simulink model "ca_interp"  (R2023b)
settings: Solver=VariableStepDiscrete  StartTime=0.0  StopTime=DUC_LINEUP_param.endTime  RelTol=1e-3  EnableMultiTasking=on
PreLoadFcn:
  | % Run the setup script when the model is opened
  | setup_ca_interp;
InitFcn:
  | % Run the setup script again just before the
  | % model is run, so that any updates made
  | % after opening are applied.
  | 
  | setup_ca_interp;
StopFcn:
  | ca_interp_output_analysis;
values from neighbouring files (symbols this model uses):
  DUC_SUMMER_multiplication_factor = 1    [setup_ca_interp.m]
  DUC_SUMMER_Number_of_bits_to_shift_left = 0    [setup_ca_interp.m]
undefined symbols (not defined in the file or in its folder): AdvDSPBChannelOutDisplay, AdvDSPBDMemDisplay, dpoly, dspba_ChannelInVis, dspba_ChannelOutVis, dspba_internal_get_channel_ports, DUC_LINEUP_param, evalAionMaskParam, latency, primtype, UseDontCare, value
libraries: DSPBAPrim x53, simulink x18, DSPBAModelBus x14, DSPBABase x12, DSPBAFilters x2
(part 1 of 2)
Description:
  | DSP Builder Advanced Template for Template Design implementing ModelIP designs
settings Model: Creator=mjervis  LastModifiedBy=5g
settings SolverCC: AlgebraicLoopSolver=TrustRegion
settings DataIOCC: LimitDataPoints=on  SaveFormat=Array  SignalLoggingSaveFormat=ModelDataLogs  ReturnWorkspaceOutputs=off
settings OptimizationCC: ExpressionDepthLimit=2147483647  LifeSpan=inf
settings DebuggingCC: UnderspecifiedInitializationDetection=Classic  MergeDetectMultiDrivingBlocksExec=none  SolverPrmCheckMsg=warning  InheritedTsInSrcMsg=none  IntegerOverflowMsg=none  FcnCallInpInsideContextMsg=warning  UnconnectedInputMsg=warning  UnconnectedOutputMsg=warning  UnconnectedLineMsg=warning  StateNameClashWarn=warning  SFUnexpectedBacktrackingDiag=warning  SFNoUnconditionalDefaultTransitionDiag=warning  SFExecutionAtInitializationDiag=none  IntegerSaturationMsg=none  ArithmeticOperatorsInVariantConditions=warning
settings HardwareCC: ProdBitPerPointer=32  ProdBitPerSizeT=32  ProdBitPerPtrDiffT=32  ProdLargestAtomicFloat=None  ProdIntDivRoundTo=Undefined  ProdEndianess=Unspecified  ProdWordSize=32  ProdHWDeviceType=32-bit Generic
settings ModelReferenceCC: EnableRefExpFcnMdlSchedulingChecks=on  PropagateSignalLabelsOutOfModel=off
settings SFSimCC: SimUseLocalCustomCode=off  CustomCodeUndefinedFunction=UseInterfaceOnly
settings RTWCC: RTWUseLocalCustomCode=off  DLArmComputeVersion=19.05
settings CodeAppCC: StateflowObjectComments=on
settings GRTTargetCC: TargetLangStandard=C89/C90 (ANSI)  CombineOutputUpdateFcns=off  GRTInterface=on
settings ConfigComp: CovMetricSettings=dw  CovSaveCumulativeToWorkspaceVar=on  CovSaveSingleToWorkspaceVar=on  CovExternalEMLEnable=off

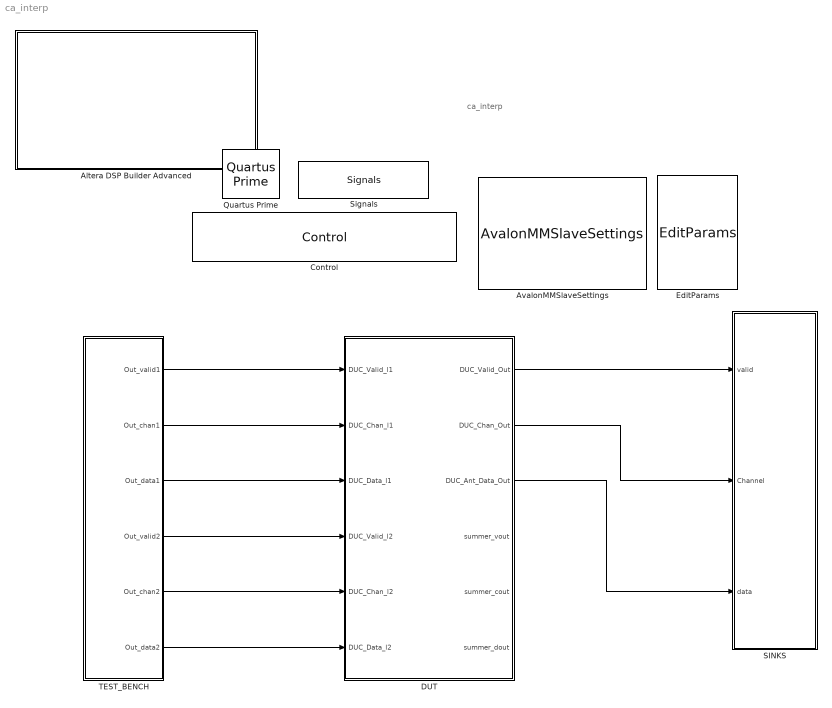
== system ca_interp ==
  note: ca_interp
  Altera DSP Builder Advanced : Subsystem  mask(DSP Builder Advanced Blockset Ignored Block){}
      settings: OpenFcn=web('http://www.altera.com', '-new');
      mask Display: image(imread('intellogo.tif'));
  AvalonMMSlaveSettings : DSPBABase/AvalonMMSlaveSettings
  Control : DSPBABase/Control  generate=on  language=VHDL  destination=./rtl  destination_gui=./rtl  make_full_path=off  path_is_relative=on  autotestbench=on  signaldepth=2  coveragetestbench=off  logs=off  spacewidth=2  spacenum=1  addrwidth=10  datawidth=16  dataendian=Big Endian  hierarchicalnames=off  ramThresholdBits=-1  distRamThresholdBits=-1  mlabThresholdBits=-1  hardMultiplierThresholdLuts=-1  version=20150801  errorOnChanMismatch=1  errorOnGPIOMismatch=0  importModelsimResults=0  cycleAccurate=off  reinterpretCastMult=off  paramFile=ca_interp_params.xml
  DUT : Subsystem
  EditParams : DSPBABase/EditParams  version=20090407
  Quartus Prime : DSPBABase/Quartus Prime  version=20090407
  SINKS : Subsystem
  Signals : DSPBABase/Signals  clk=clk  freq=240  margin=0  rst=areset  rstactive=High  bus=bus  enbusclock=off  busfreq=491.52  bussync=off  version=20090407
  TEST_BENCH : Subsystem
  wires:
  DUT/1(DUC_Valid_Out) -> SINKS/1(valid)
  DUT/3(DUC_Ant_Data_Out) -> SINKS/3(data)
  DUT/2(DUC_Chan_Out) -> SINKS/2(Channel)
  TEST_BENCH/1(Out_valid1) -> DUT/1(DUC_Valid_l1)
  TEST_BENCH/2(Out_chan1) -> DUT/2(DUC_Chan_l1)
  TEST_BENCH/3(Out_data1) -> DUT/3(DUC_Data_l1)
  TEST_BENCH/4(Out_valid2) -> DUT/4(DUC_Valid_l2)
  TEST_BENCH/5(Out_chan2) -> DUT/5(DUC_Chan_l2)
  TEST_BENCH/6(Out_data2) -> DUT/6(DUC_Data_l2)

== system ca_interp/Altera DSP Builder Advanced ==

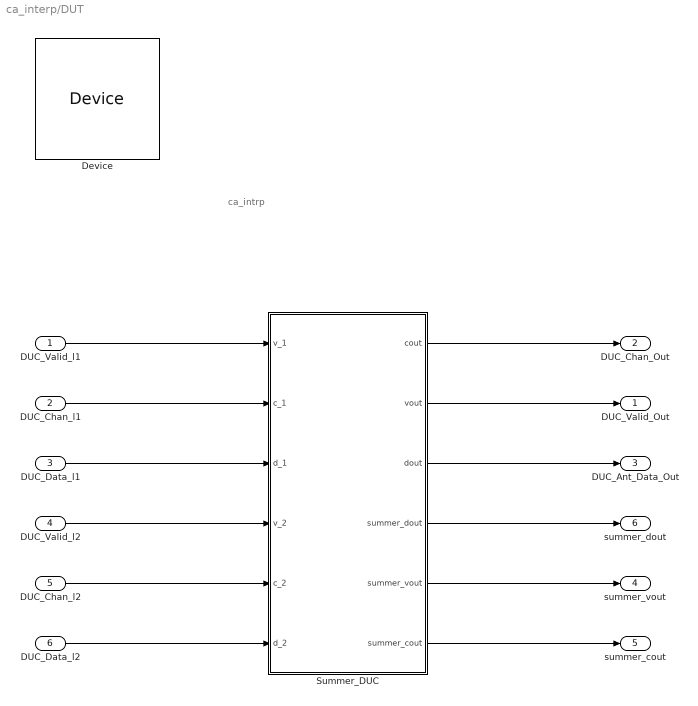
== system ca_interp/DUT ==
  note: ca_intrp
  DUC_Valid_l1 : Inport
  DUC_Chan_l1 : Inport  Port=2
  DUC_Data_l1 : Inport  Port=3
  DUC_Valid_l2 : Inport  Port=4
  DUC_Chan_l2 : Inport  Port=5
  DUC_Data_l2 : Inport  Port=6
  Device : DSPBABase/Device  family=Arria 10  deviceMember=Stratix V GX  stratix4device=Stratix IV GX  hardcopy4device=HardCopy IV E  stratix5device=Stratix V GX  device=10AS066N2F40I1SGES  speed=1  stratixSpeed=-5  stratix2Speed=-3  stratix3Speed=-3  stratix4gxSpeed=-2  stratix4gtSpeed=-1  cyclone2Speed=-6  cyclone3Speed=-7  arria2Speed=-4  cyclone4eSpeed=-8  stratix5Speed=-3  arria5Speed=-4  arriaSpeed=-6  cyclone3lsSpeed=-7  cyclone5Speed=-6  arria2gzSpeed=-3  nightFurySpeed=-2  ecp2Speed=-7  hardcopycompat=off  version=20140217  max10flashmode=off  max10nomeminit=off
  Summer_DUC : Subsystem
  DUC_Valid_Out : Outport
  DUC_Chan_Out : Outport  Port=2
  DUC_Ant_Data_Out : Outport  Port=3
  summer_vout : Outport  Port=4
  summer_cout : Outport  Port=5
  summer_dout : Outport  Port=6
  wires:
  DUC_Valid_l2/1 -> Summer_DUC/4(v_2)
  DUC_Chan_l2/1 -> Summer_DUC/5(c_2)
  DUC_Data_l2/1 -> Summer_DUC/6(d_2)
  DUC_Valid_l1/1 -> Summer_DUC/1(v_1)
  DUC_Chan_l1/1 -> Summer_DUC/2(c_1)
  DUC_Data_l1/1 -> Summer_DUC/3(d_1)
  Summer_DUC/3(dout) -> DUC_Ant_Data_Out/1
  Summer_DUC/2(vout) -> DUC_Valid_Out/1
  Summer_DUC/1(cout) -> DUC_Chan_Out/1
  Summer_DUC/4(summer_dout) -> summer_dout/1
  Summer_DUC/5(summer_vout) -> summer_vout/1
  Summer_DUC/6(summer_cout) -> summer_cout/1

== system ca_interp/SINKS ==
  valid : Inport
  Channel : Inport  Port=2
  data : Inport  Port=3
  ChanView : DSPBABase/ChanView  nchans=8  chan_vector=[0:7]  outsvalid=off  latency=1  version=20090407
  ChanView1 : DSPBABase/ChanView  nchans=8  chan_vector=[0:7]  outsvalid=off  latency=1  version=20090407
  Complex to Real-Imag2 : ComplexToRealImag
  ImagScope : Scope  NumInputPorts=8
  RealScope : Scope  NumInputPorts=8
  Scope : Scope  NumInputPorts=3
  To Workspace : ToWorkspace  Commented=on  VariableName=DUC_Ant_Data_out  SaveFormat=Timeseries  SampleTime=-1
  To Workspace1 : ToWorkspace  Commented=on  VariableName=DUC_Ant_Data_vout  SaveFormat=Timeseries  SampleTime=-1
  TraceAntennaData : Subsystem  Commented=on  TreatAsAtomicUnit=on
  TraceAntennaData1 : Subsystem  TreatAsAtomicUnit=on
  dataScope : Scope  NumInputPorts=2
  wires:
  Complex to Real-Imag2/1 -> dataScope/1, ChanView/1
  Channel/1 -> TraceAntennaData1/2(ChIn), Scope/2, ChanView1/3, ChanView/3
  Complex to Real-Imag2/2 -> dataScope/2, ChanView1/1
  ChanView1/2 -> ImagScope/2
  ChanView1/3 -> ImagScope/3
  ChanView1/4 -> ImagScope/4
  ChanView1/1 -> ImagScope/1
  ChanView/3 -> RealScope/3
  ChanView/1 -> RealScope/1
  ChanView/4 -> RealScope/4
  ChanView/2 -> RealScope/2
  ChanView/5 -> RealScope/5
  ChanView/6 -> RealScope/6
  ChanView/7 -> RealScope/7
  ChanView/8 -> RealScope/8
  ChanView1/5 -> ImagScope/5
  ChanView1/6 -> ImagScope/6
  ChanView1/7 -> ImagScope/7
  ChanView1/8 -> ImagScope/8
  valid/1 -> TraceAntennaData1/Enable, To Workspace1/1, Scope/1, TraceAntennaData/Enable, ChanView1/2, ChanView/2
  data/1 -> TraceAntennaData1/1(DataIn), To Workspace/1, Scope/3, TraceAntennaData/1(DataIn), Complex to Real-Imag2/1

== system ca_interp/TEST_BENCH ==
  Data Type Conversion : DataTypeConversion  OutDataTypeStr=uint8  SaturateOnIntegerOverflow=off  RndMeth=Floor
  Repeating Sequence channel : simulink/Sources/Repeating Sequence Stair  OutValues=DUC_LINEUP_param.duc_channel  tsamp=1  OutMin=[]  OutMax=[]  OutDataTypeStr=uint8  OutputDataTypeScalingMode=uint8  OutDataType=fixdt(1,16)  ConRadixGroup=Best Precision: Vector-wise  OutScaling=[]
  Repeating Sequence valid : simulink/Sources/Repeating Sequence Stair  OutValues=DUC_LINEUP_param.duc_valid  tsamp=1  OutMin=[]  OutMax=[]  OutDataTypeStr=fixdt('boolean')  OutputDataTypeScalingMode=Specify via dialog  OutDataType=fixdt('boolean')  ConRadixGroup=Best Precision: Vector-wise  OutScaling=[]
  Subsystem1 : Subsystem
  Subsystem2 : Subsystem
  Out_valid1 : Outport
  Out_chan1 : Outport  Port=2
  Out_data1 : Outport  Port=3
  Out_valid2 : Outport  Port=4
  Out_chan2 : Outport  Port=5
  Out_data2 : Outport  Port=6
  wires:
  Repeating Sequence valid/1 -> Out_valid2/1, Out_valid1/1  "valid signal"
  Repeating Sequence channel/1 -> Data Type Conversion/1  "channel count signal"
  Data Type Conversion/1 -> Out_chan2/1, Out_chan1/1
  Subsystem1/1(Out_data1) -> Out_data1/1
  Subsystem2/1(Out_data2) -> Out_data2/1

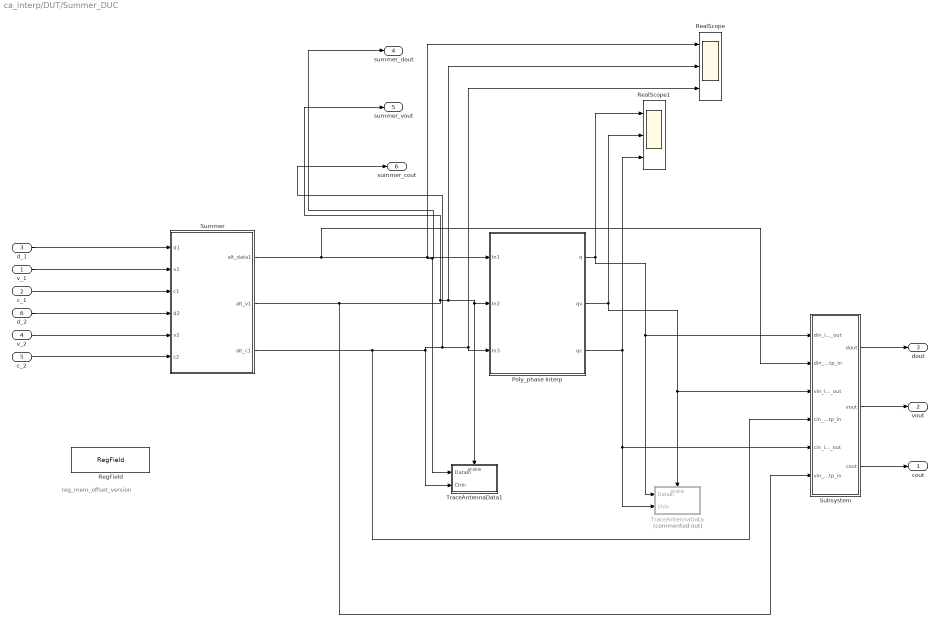
== system ca_interp/DUT/Summer_DUC ==
  note: reg_mem_offset_version
  v_1 : Inport
  c_1 : Inport  Port=2
  d_1 : Inport  Port=3
  v_2 : Inport  Port=4
  c_2 : Inport  Port=5
  d_2 : Inport  Port=6
  Poly_phase Interp : Subsystem
  RealScope : Scope  NumInputPorts=3
  RealScope1 : Scope  NumInputPorts=3
  RegField : DSPBAModelBus/RegField  reg_name=DUC_LINEUP_param.reg_version.mem_offset  reg_rwmode=Read/Write  reg_msb=31  reg_lsb=0  reg_mode=Specify via dialog  reg_type=ufix(32)  reg_scale=2^0  reg_init=DUC_LINEUP_param.reg_version.Version_reg_val  reg_desc=Version_Output  reg_modal=off  reg_desc0=0  reg_desc1=0  reg_desc2=0  reg_desc3=0  reg_desc4=0  reg_desc5=0  reg_desc6=0  reg_desc7=0  reg_addr=13  SampleTime=-1  version=20090407
  Subsystem : Subsystem
  Summer : Subsystem  mask{ClockMargin=DUC_LINEUP_param.ClockMargin, output_word_length=DUC_LINEUP_param.output_word_length, output_fraction_length=DUC_LINEUP_param.output_fraction_length, Summer_Multiplication_fact=DUC_SUMMER_multiplication_factor, Summer_left_shift_fact=DUC_SUMMER_Number_of_bits_to_shift_left, Pipeline_stages=2}
      mask Display:
      | disp('SUMMER');
      | port_label('input',1,'d0');
      | port_label('input',2,'v0');
      | port_label('input',3,'c0');
      | 
      | port_label('input',4,'d1');
      | port_label('input',5,'v1');
      | port_label('input',6,'c1');
      | 
      | 
      | port_label('output',1,'q');
      | port_label('output',2,'q_v');
      | port_label('output',3,'q_c');
  TraceAntennaData : Subsystem  Commented=on  TreatAsAtomicUnit=on
  TraceAntennaData1 : Subsystem  TreatAsAtomicUnit=on
  cout : Outport
  vout : Outport  Port=2
  dout : Outport  Port=3
  summer_dout : Outport  Port=4
  summer_vout : Outport  Port=5
  summer_cout : Outport  Port=6
  wires:
  c_1/1 -> Summer/3(c1)
  d_2/1 -> Summer/4(d2)
  v_2/1 -> Summer/5(v2)
  c_2/1 -> Summer/6(c2)
  v_1/1 -> Summer/2(v1)
  d_1/1 -> Summer/1(d1)
  Summer/2(alt_v1) -> Subsystem/6(vin_intp_in), summer_vout/1, TraceAntennaData1/Enable, Poly_phase Interp/2(In2), RealScope/2
  Summer/3(alt_c1) -> Subsystem/4(cin_intp_in), summer_cout/1, RealScope/3, Poly_phase Interp/3(In3), TraceAntennaData1/2(ChIn)
  Poly_phase Interp/1(q) -> RealScope1/1, TraceAntennaData/1(DataIn), Subsystem/1(din_intp_out)
  Poly_phase Interp/2(qv) -> RealScope1/2, Subsystem/3(vin_intp_out), TraceAntennaData/Enable
  Poly_phase Interp/3(qc) -> RealScope1/3, TraceAntennaData/2(ChIn), Subsystem/5(cin_intp_out)
  Summer/1(alt_data1) -> RealScope/1, Poly_phase Interp/1(In1), summer_dout/1, TraceAntennaData1/1(DataIn), Subsystem/2(din_intp_in)
  Subsystem/1(dout) -> dout/1
  Subsystem/2(vout) -> vout/1
  Subsystem/3(cout) -> cout/1

== system ca_interp/SINKS/TraceAntennaData ==
  DataIn : Inport
  Enable : EnablePort
  DucAntDataOut : ToWorkspace  VariableName=DUC_Ant_Data_Out  SaveFormat=Timeseries  SampleTime=-1
  wires:
  DataIn/1 -> DucAntDataOut/1

== system ca_interp/SINKS/TraceAntennaData1 ==
  DataIn : Inport
  ChIn : Inport  Port=2
  Enable : EnablePort
  DucAntDataOut : ToWorkspace  VariableName=PolyPhase0_dOut  SampleTime=-1
  DucAntDataOut1 : ToWorkspace  VariableName=PolyPhase0_cOut  SampleTime=-1
  wires:
  DataIn/1 -> DucAntDataOut/1
  ChIn/1 -> DucAntDataOut1/1

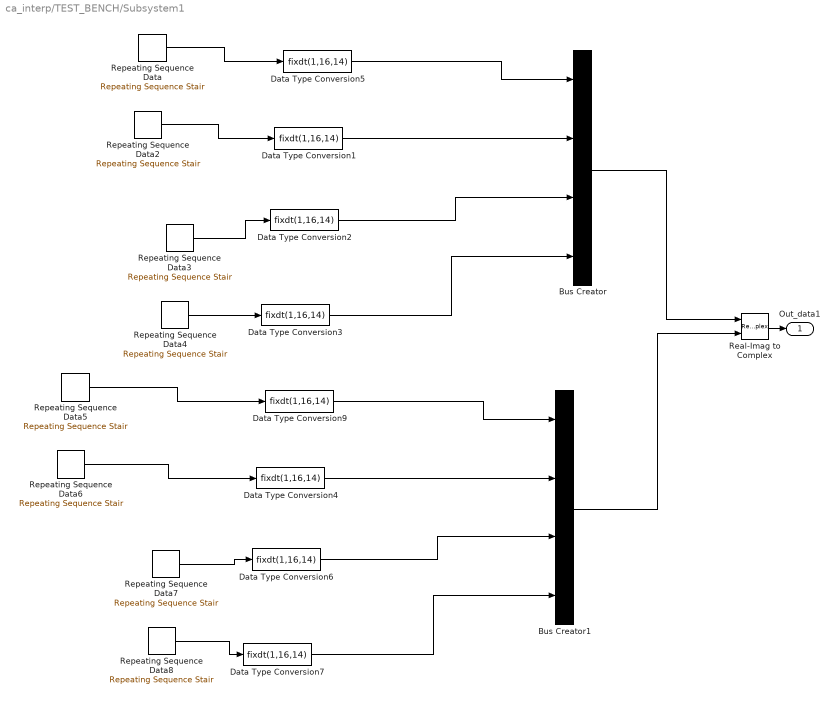
== system ca_interp/TEST_BENCH/Subsystem1 ==
  Bus Creator : BusCreator  Inputs=4
  Bus Creator1 : BusCreator  Inputs=4
  Data Type Conversion{1..7,9} (8 alike) : DataTypeConversion  OutDataTypeStr=fixdt(1,16,14)  SaturateOnIntegerOverflow=off  RndMeth=Floor
  Real-Imag to Complex : RealImagToComplex
  Repeating Sequence Data : simulink/Sources/Repeating Sequence Stair  OutValues=real(DUC_LINEUP_param.inputdata_l1(:,1))  tsamp=1  OutMin=[]  OutMax=[]  OutDataTypeStr=fixdt(1,16)  OutputDataTypeScalingMode=Specify via dialog  OutDataType=fixdt(1,16)  ConRadixGroup=Best Precision: Vector-wise  OutScaling=[]
  Repeating Sequence Data2 : simulink/Sources/Repeating Sequence Stair  OutValues=real(DUC_LINEUP_param.inputdata_l1(:,2))  tsamp=1  OutMin=[]  OutMax=[]  OutDataTypeStr=fixdt(1,16)  OutputDataTypeScalingMode=Specify via dialog  OutDataType=fixdt(1,16)  ConRadixGroup=Best Precision: Vector-wise  OutScaling=[]
  Repeating Sequence Data3 : simulink/Sources/Repeating Sequence Stair  OutValues=real(DUC_LINEUP_param.inputdata_l1(:,3))  tsamp=1  OutMin=[]  OutMax=[]  OutDataTypeStr=fixdt(1,16)  OutputDataTypeScalingMode=Specify via dialog  OutDataType=fixdt(1,16)  ConRadixGroup=Best Precision: Vector-wise  OutScaling=[]
  Repeating Sequence Data4 : simulink/Sources/Repeating Sequence Stair  OutValues=real(DUC_LINEUP_param.inputdata_l1(:,4))  tsamp=1  OutMin=[]  OutMax=[]  OutDataTypeStr=fixdt(1,16)  OutputDataTypeScalingMode=Specify via dialog  OutDataType=fixdt(1,16)  ConRadixGroup=Best Precision: Vector-wise  OutScaling=[]
  Repeating Sequence Data5 : simulink/Sources/Repeating Sequence Stair  OutValues=imag(DUC_LINEUP_param.inputdata_l1(:,1))  tsamp=1  OutMin=[]  OutMax=[]  OutDataTypeStr=fixdt(1,16)  OutputDataTypeScalingMode=Specify via dialog  OutDataType=fixdt(1,16)  ConRadixGroup=Best Precision: Vector-wise  OutScaling=[]
  Repeating Sequence Data6 : simulink/Sources/Repeating Sequence Stair  OutValues=imag(DUC_LINEUP_param.inputdata_l1(:,2))  tsamp=1  OutMin=[]  OutMax=[]  OutDataTypeStr=fixdt(1,16)  OutputDataTypeScalingMode=Specify via dialog  OutDataType=fixdt(1,16)  ConRadixGroup=Best Precision: Vector-wise  OutScaling=[]
  Repeating Sequence Data7 : simulink/Sources/Repeating Sequence Stair  OutValues=imag(DUC_LINEUP_param.inputdata_l1(:,3))  tsamp=1  OutMin=[]  OutMax=[]  OutDataTypeStr=fixdt(1,16)  OutputDataTypeScalingMode=Specify via dialog  OutDataType=fixdt(1,16)  ConRadixGroup=Best Precision: Vector-wise  OutScaling=[]
  Repeating Sequence Data8 : simulink/Sources/Repeating Sequence Stair  OutValues=imag(DUC_LINEUP_param.inputdata_l1(:,4))  tsamp=1  OutMin=[]  OutMax=[]  OutDataTypeStr=fixdt(1,16)  OutputDataTypeScalingMode=Specify via dialog  OutDataType=fixdt(1,16)  ConRadixGroup=Best Precision: Vector-wise  OutScaling=[]
  Out_data1 : Outport
  wires:
  Data Type Conversion6/1 -> Bus Creator1/3
  Bus Creator1/1 -> Real-Imag to Complex/2
  Repeating Sequence Data/1 -> Data Type Conversion5/1
  Data Type Conversion3/1 -> Bus Creator/4
  Repeating Sequence Data8/1 -> Data Type Conversion7/1
  Data Type Conversion5/1 -> Bus Creator/1
  Real-Imag to Complex/1 -> Out_data1/1
  Repeating Sequence Data2/1 -> Data Type Conversion1/1
  Bus Creator/1 -> Real-Imag to Complex/1
  Data Type Conversion9/1 -> Bus Creator1/1
  Data Type Conversion1/1 -> Bus Creator/2
  Repeating Sequence Data3/1 -> Data Type Conversion2/1
  Repeating Sequence Data7/1 -> Data Type Conversion6/1
  Repeating Sequence Data4/1 -> Data Type Conversion3/1
  Repeating Sequence Data6/1 -> Data Type Conversion4/1
  Data Type Conversion2/1 -> Bus Creator/3
  Repeating Sequence Data5/1 -> Data Type Conversion9/1
  Data Type Conversion7/1 -> Bus Creator1/4
  Data Type Conversion4/1 -> Bus Creator1/2

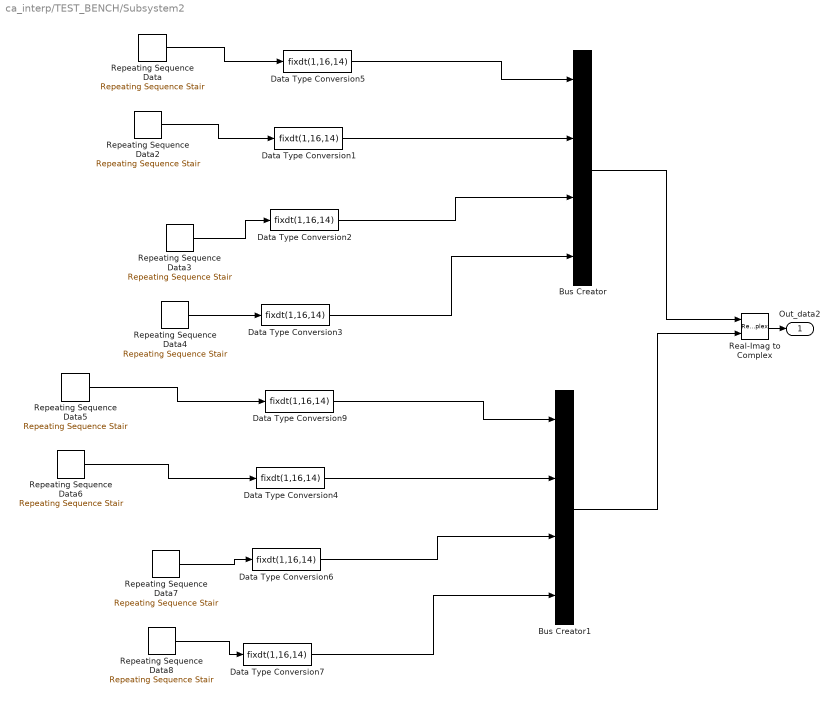
== system ca_interp/TEST_BENCH/Subsystem2 ==
  Bus Creator : BusCreator  Inputs=4
  Bus Creator1 : BusCreator  Inputs=4
  Data Type Conversion{1..7,9} (8 alike) : DataTypeConversion  OutDataTypeStr=fixdt(1,16,14)  SaturateOnIntegerOverflow=off  RndMeth=Floor
  Real-Imag to Complex : RealImagToComplex
  Repeating Sequence Data : simulink/Sources/Repeating Sequence Stair  OutValues=real(DUC_LINEUP_param.inputdata_l2(:,1))  tsamp=1  OutMin=[]  OutMax=[]  OutDataTypeStr=fixdt(1,16)  OutputDataTypeScalingMode=Specify via dialog  OutDataType=fixdt(1,16)  ConRadixGroup=Best Precision: Vector-wise  OutScaling=[]
  Repeating Sequence Data2 : simulink/Sources/Repeating Sequence Stair  OutValues=real(DUC_LINEUP_param.inputdata_l2(:,2))  tsamp=1  OutMin=[]  OutMax=[]  OutDataTypeStr=fixdt(1,16)  OutputDataTypeScalingMode=Specify via dialog  OutDataType=fixdt(1,16)  ConRadixGroup=Best Precision: Vector-wise  OutScaling=[]
  Repeating Sequence Data3 : simulink/Sources/Repeating Sequence Stair  OutValues=real(DUC_LINEUP_param.inputdata_l2(:,3))  tsamp=1  OutMin=[]  OutMax=[]  OutDataTypeStr=fixdt(1,16)  OutputDataTypeScalingMode=Specify via dialog  OutDataType=fixdt(1,16)  ConRadixGroup=Best Precision: Vector-wise  OutScaling=[]
  Repeating Sequence Data4 : simulink/Sources/Repeating Sequence Stair  OutValues=real(DUC_LINEUP_param.inputdata_l2(:,4))  tsamp=1  OutMin=[]  OutMax=[]  OutDataTypeStr=fixdt(1,16)  OutputDataTypeScalingMode=Specify via dialog  OutDataType=fixdt(1,16)  ConRadixGroup=Best Precision: Vector-wise  OutScaling=[]
  Repeating Sequence Data5 : simulink/Sources/Repeating Sequence Stair  OutValues=imag(DUC_LINEUP_param.inputdata_l2(:,1))  tsamp=1  OutMin=[]  OutMax=[]  OutDataTypeStr=fixdt(1,16)  OutputDataTypeScalingMode=Specify via dialog  OutDataType=fixdt(1,16)  ConRadixGroup=Best Precision: Vector-wise  OutScaling=[]
  Repeating Sequence Data6 : simulink/Sources/Repeating Sequence Stair  OutValues=imag(DUC_LINEUP_param.inputdata_l2(:,2))  tsamp=1  OutMin=[]  OutMax=[]  OutDataTypeStr=fixdt(1,16)  OutputDataTypeScalingMode=Specify via dialog  OutDataType=fixdt(1,16)  ConRadixGroup=Best Precision: Vector-wise  OutScaling=[]
  Repeating Sequence Data7 : simulink/Sources/Repeating Sequence Stair  OutValues=imag(DUC_LINEUP_param.inputdata_l2(:,3))  tsamp=1  OutMin=[]  OutMax=[]  OutDataTypeStr=fixdt(1,16)  OutputDataTypeScalingMode=Specify via dialog  OutDataType=fixdt(1,16)  ConRadixGroup=Best Precision: Vector-wise  OutScaling=[]
  Repeating Sequence Data8 : simulink/Sources/Repeating Sequence Stair  OutValues=imag(DUC_LINEUP_param.inputdata_l2(:,4))  tsamp=1  OutMin=[]  OutMax=[]  OutDataTypeStr=fixdt(1,16)  OutputDataTypeScalingMode=Specify via dialog  OutDataType=fixdt(1,16)  ConRadixGroup=Best Precision: Vector-wise  OutScaling=[]
  Out_data2 : Outport
  wires:
  Data Type Conversion4/1 -> Bus Creator1/2
  Data Type Conversion7/1 -> Bus Creator1/4
  Repeating Sequence Data5/1 -> Data Type Conversion9/1
  Data Type Conversion2/1 -> Bus Creator/3
  Repeating Sequence Data6/1 -> Data Type Conversion4/1
  Repeating Sequence Data4/1 -> Data Type Conversion3/1
  Repeating Sequence Data7/1 -> Data Type Conversion6/1
  Repeating Sequence Data3/1 -> Data Type Conversion2/1
  Data Type Conversion1/1 -> Bus Creator/2
  Data Type Conversion9/1 -> Bus Creator1/1
  Bus Creator/1 -> Real-Imag to Complex/1
  Repeating Sequence Data2/1 -> Data Type Conversion1/1
  Real-Imag to Complex/1 -> Out_data2/1
  Data Type Conversion5/1 -> Bus Creator/1
  Repeating Sequence Data8/1 -> Data Type Conversion7/1
  Data Type Conversion3/1 -> Bus Creator/4
  Repeating Sequence Data/1 -> Data Type Conversion5/1
  Bus Creator1/1 -> Real-Imag to Complex/2
  Data Type Conversion6/1 -> Bus Creator1/3

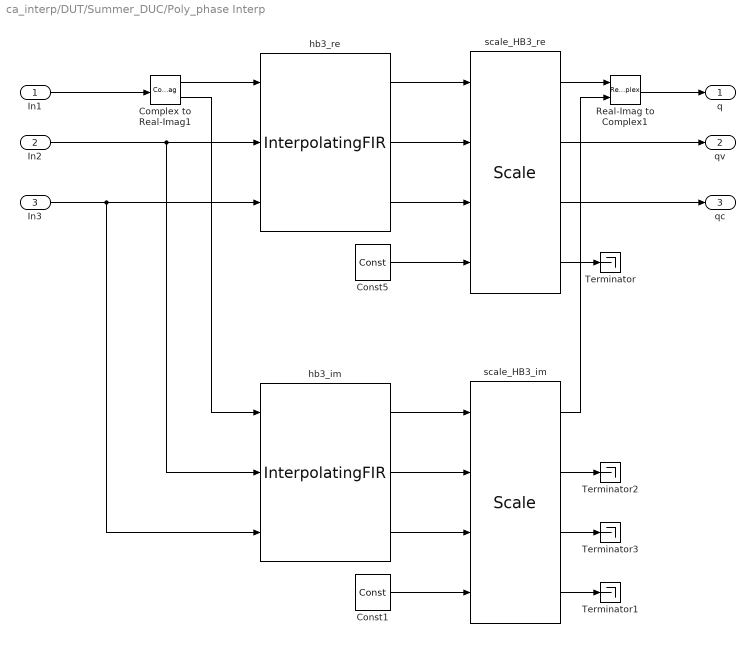
== system ca_interp/DUT/Summer_DUC/Poly_phase Interp ==
  In1 : Inport
  In2 : Inport  Port=2
  In3 : Inport  Port=3
  Complex to Real-Imag1 : ComplexToRealImag
  Const1 : DSPBAPrim/Const  primtype=const  nInputs=0  nOutputs=1  omode=Inherit via internal rule  otype=sfix(16)  scale=2^-15  rndmethod=Unbiased  factor=1  satmethod=Symmetric  shift_vec=[0 1 2 -1]  value=0  inPortNames=['+'; '+';]  outPortNames=[' ']  dspbaimage=dspba_prim.svg  text=fprintf('%s', num2str(value));  style=Optimised  visibilities=8 + 1024  floatPrecision=float32_m23  warnSaturation=on  version=20211007  SampleTime=inf
  Const5 : DSPBAPrim/Const  primtype=const  nInputs=0  nOutputs=1  omode=Inherit via internal rule  otype=sfix(16)  scale=2^-15  rndmethod=Unbiased  factor=1  satmethod=Symmetric  shift_vec=[0 1 2 -1]  value=0  inPortNames=['+'; '+';]  outPortNames=[' ']  dspbaimage=dspba_prim.svg  text=fprintf('%s', num2str(value));  style=Optimised  visibilities=8 + 1024  floatPrecision=float32_m23  warnSaturation=on  version=20211007  SampleTime=inf
  Real-Imag to Complex1 : RealImagToComplex
  Terminator{,1..3} (4 alike) : Terminator
  hb3_im : DSPBAFilters/InterpolatingFIR  nInputRate=491.52  interp=2  nchan=DUC_LINEUP_param.ChanCount  symmetry=Symmetrical  coef=DUC_LINEUP_param.HB_filt3.coeffs  addr=DUC_LINEUP_param.HB_filt6.base_addr_l3  rwmode=Constant  nband=Half Band  exposebus=off  latency=5  version=20090407  recon=off  MM=[0,1,2,3,4,5,6,7,8,9,10,11,12,13,14,15]  resetrezero=off  sharecoef=auto  simulationMode=Standard
  hb3_re : DSPBAFilters/InterpolatingFIR  nInputRate=491.52  interp=2  nchan=DUC_LINEUP_param.ChanCount  symmetry=Symmetrical  coef=DUC_LINEUP_param.HB_filt3.coeffs  addr=DUC_LINEUP_param.HB_filt6.base_addr_l3  rwmode=Constant  nband=Half Band  exposebus=off  latency=5  version=20090407  recon=off  MM=[0,1,2,3,4,5,6,7,8,9,10,11,12,13,14,15]  resetrezero=off  sharecoef=auto  simulationMode=Standard
  scale_HB3_im : DSPBABase/Scale  otype=sfix(DUC_LINEUP_param.output_word_length)  scale=2^-DUC_LINEUP_param.output_fraction_length  rndmethod=Biased  factor=1  satmethod=None  shift_vec=1  latency=2  simulationMode=Use Global Value  version=20090407
  scale_HB3_re : DSPBABase/Scale  otype=sfix(DUC_LINEUP_param.output_word_length)  scale=2^-DUC_LINEUP_param.output_fraction_length  rndmethod=Biased  factor=1  satmethod=None  shift_vec=1  latency=2  simulationMode=Use Global Value  version=20090407
  q : Outport
  qv : Outport  Port=2
  qc : Outport  Port=3
  wires:
  scale_HB3_im/4 -> Terminator1/1
  In3/1 -> hb3_im/3, hb3_re/3
  Complex to Real-Imag1/1 -> hb3_re/1
  hb3_im/1 -> scale_HB3_im/1
  Complex to Real-Imag1/2 -> hb3_im/1
  In1/1 -> Complex to Real-Imag1/1
  hb3_re/2 -> scale_HB3_re/2
  scale_HB3_re/1 -> Real-Imag to Complex1/1
  scale_HB3_im/2 -> Terminator2/1
  scale_HB3_im/1 -> Real-Imag to Complex1/2
  Const1/1 -> scale_HB3_im/4
  Const5/1 -> scale_HB3_re/4
  scale_HB3_im/3 -> Terminator3/1
  scale_HB3_re/4 -> Terminator/1
  hb3_re/1 -> scale_HB3_re/1
  scale_HB3_re/3 -> qc/1
  hb3_im/3 -> scale_HB3_im/3
  hb3_re/3 -> scale_HB3_re/3
  scale_HB3_re/2 -> qv/1
  hb3_im/2 -> scale_HB3_im/2
  Real-Imag to Complex1/1 -> q/1
  In2/1 -> hb3_im/2, hb3_re/2

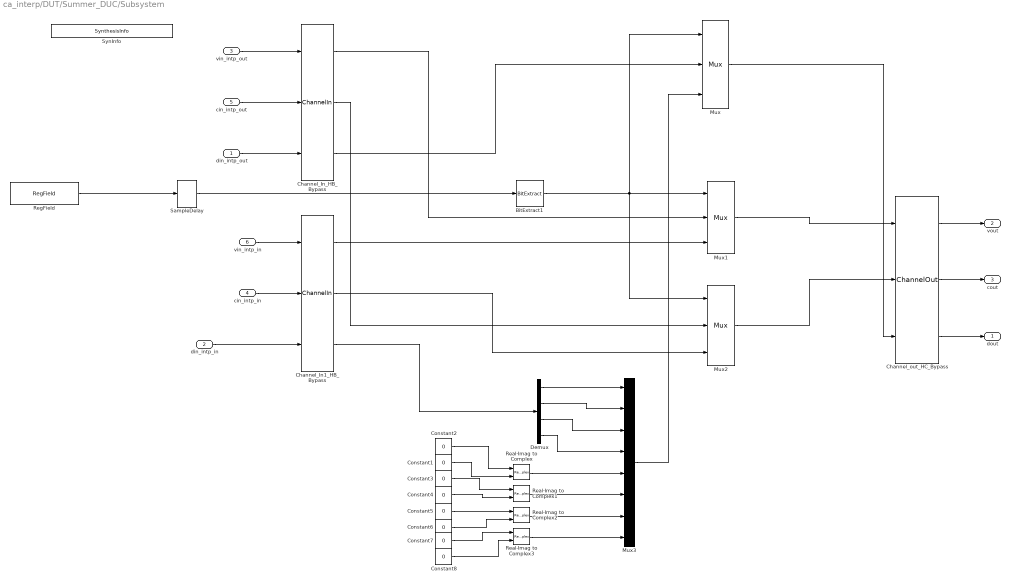
== system ca_interp/DUT/Summer_DUC/Subsystem ==
  din_intp_out : Inport
  din_intp_in : Inport  Port=2
  vin_intp_out : Inport  Port=3
  cin_intp_in : Inport  Port=4
  cin_intp_out : Inport  Port=5
  vin_intp_in : Inport  Port=6
  BitExtract1 : DSPBAPrim/BitExtract  primtype=bitextract  nInputs=1  nOutputs=1  omode=boolean  otype=uint(16)  scale=1  rndmethod=Unbiased  factor=1  satmethod=Symmetric  shift_vec=[0 1 2 -1]  value=0  inPortNames=[' '; ' ';]  outPortNames=[' ']  dspbaimage=dspba_prim.svg  text=fprintf('..%d', value);  style=Optimised  visibilities=8+1024  version=20211007
  Channel_In1_HB_Bypass : DSPBAPrim/ChannelIn  primtype=channelin  nInputs=dspba_internal_get_channel_ports(gcb)  nOutputs=dspba_internal_get_channel_ports(gcb)  omode=Inherit via internal rule  otype=sfix(16)  scale=2^-15  rndmethod=Unbiased  factor=1  satmethod=Symmetric  shift_vec=[0 1 2 -1]  value=1  inPortNames=['v'; 'c'; '0'; '1'; '2'; '3'; '4'; '5'; '6'; '7'; '8'; '9'; 'A'; 'B'; 'D'; 'E'; 'F'; 'G'; 'H'; 'I'; 'J'; 'K'; 'L'; 'M'; 'N'; 'O'; 'P'; 'Q'; 'R'; 'S'; 'T'; 'U'; 'W'; 'X'; 'Y'; 'Z']  outPortNames=['v'; 'c'; '0'; '1'; '2'; '3'; '4'; '5'; '6'; '7'; '8'; '9'; 'A'; 'B'; 'D'; 'E'; 'F'; 'G'; 'H'; 'I'; 'J'; 'K'; 'L'; 'M'; 'N'; 'O'; 'P'; 'Q'; 'R'; 'S'; 'T'; 'U'; 'W'; 'X'; 'Y'; 'Z']  dspbaimage=dspba_prim_channel_tall.svg  text=fprintf('In');  style=Optimised  dataSignals=1  foldingEnabled=off  channels=1  sampleRate=200  packetBeginPresent=off  packetBeginEnabled=off  visibilities=dspba_ChannelInVis(gcb)  scheduleOrigin=on  version=20211214
  Channel_In_HB_Bypass : DSPBAPrim/ChannelIn  primtype=channelin  nInputs=dspba_internal_get_channel_ports(gcb)  nOutputs=dspba_internal_get_channel_ports(gcb)  omode=Inherit via internal rule  otype=sfix(16)  scale=2^-15  rndmethod=Unbiased  factor=1  satmethod=Symmetric  shift_vec=[0 1 2 -1]  value=1  inPortNames=['v'; 'c'; '0'; '1'; '2'; '3'; '4'; '5'; '6'; '7'; '8'; '9'; 'A'; 'B'; 'D'; 'E'; 'F'; 'G'; 'H'; 'I'; 'J'; 'K'; 'L'; 'M'; 'N'; 'O'; 'P'; 'Q'; 'R'; 'S'; 'T'; 'U'; 'W'; 'X'; 'Y'; 'Z']  outPortNames=['v'; 'c'; '0'; '1'; '2'; '3'; '4'; '5'; '6'; '7'; '8'; '9'; 'A'; 'B'; 'D'; 'E'; 'F'; 'G'; 'H'; 'I'; 'J'; 'K'; 'L'; 'M'; 'N'; 'O'; 'P'; 'Q'; 'R'; 'S'; 'T'; 'U'; 'W'; 'X'; 'Y'; 'Z']  dspbaimage=dspba_prim_channel_tall.svg  text=fprintf('In');  style=Optimised  dataSignals=1  foldingEnabled=off  channels=1  sampleRate=200  packetBeginPresent=off  packetBeginEnabled=off  visibilities=dspba_ChannelInVis(gcb)  scheduleOrigin=on  version=20211214
  Channel_out_HC_Bypass : DSPBAPrim/ChannelOut  primtype=channelout  nInputs=dspba_internal_get_channel_ports(gcb)  nOutputs=dspba_internal_get_channel_ports(gcb)  omode=Inherit via internal rule  otype=sfix(16)  scale=2^-15  rndmethod=Unbiased  factor=1  satmethod=Symmetric  shift_vec=[0 1 2 -1]  value=1  inPortNames=['v'; 'c'; '0'; '1'; '2'; '3'; '4'; '5'; '6'; '7'; '8'; '9'; 'A'; 'B'; 'D'; 'E'; 'F'; 'G'; 'H'; 'I'; 'J'; 'K'; 'L'; 'M'; 'N'; 'O'; 'P'; 'Q'; 'R'; 'S'; 'T'; 'U'; 'W'; 'X'; 'Y'; 'Z']  outPortNames=['v'; 'c'; '0'; '1'; '2'; '3'; '4'; '5'; '6'; '7'; '8'; '9'; 'A'; 'B'; 'D'; 'E'; 'F'; 'G'; 'H'; 'I'; 'J'; 'K'; 'L'; 'M'; 'N'; 'O'; 'P'; 'Q'; 'R'; 'S'; 'T'; 'U'; 'W'; 'X'; 'Y'; 'Z']  dspbaimage=dspba_prim_channel_tall.svg  text=fprintf('Out%s', AdvDSPBChannelOutDisplay(latency));  style=Optimised  dataSignals=1  foldingEnabled=off  channels=1  sampleRate=200  packetBeginPresent=off  packetBeginEnabled=off  visibilities=dspba_ChannelOutVis(gcb)  latency=0  version=20211214
  Constant{1..8} (8 alike) : Constant  Value=0  OutDataTypeStr=fixdt(1,DUC_LINEUP_param.output_word_length ,DUC_LINEUP_param.output_fraction_length)
  Demux : Demux
  Mux : DSPBAPrim/Mux  primtype=mux  nInputs=evalAionMaskParam(gcb,'value',1)+1  nOutputs=1  omode=Inherit via internal rule  otype=sfix(16)  scale=2^-15  rndmethod=Unbiased  factor=1  satmethod=Symmetric  shift_vec=[0 1 2 -1]  value=2  inPortNames=['s '; 'd0'; 'd1'; 'd2'; 'd3'; 'd4'; 'd5'; 'd6'; 'd7'; 'd8'; 'd9';]  outPortNames=[' ']  dspbaimage=dspba_prim_tall.svg  text=fprintf('%s', primtype);  style=Optimised  visibilities=1032  version=20211007
  Mux1 : DSPBAPrim/Mux  primtype=mux  nInputs=evalAionMaskParam(gcb,'value',1)+1  nOutputs=1  omode=Inherit via internal rule  otype=sfix(16)  scale=2^-15  rndmethod=Unbiased  factor=1  satmethod=Symmetric  shift_vec=[0 1 2 -1]  value=2  inPortNames=['s '; 'd0'; 'd1'; 'd2'; 'd3'; 'd4'; 'd5'; 'd6'; 'd7'; 'd8'; 'd9';]  outPortNames=[' ']  dspbaimage=dspba_prim_tall.svg  text=fprintf('%s', primtype);  style=Optimised  visibilities=1032  version=20211007
  Mux2 : DSPBAPrim/Mux  primtype=mux  nInputs=evalAionMaskParam(gcb,'value',1)+1  nOutputs=1  omode=Inherit via internal rule  otype=sfix(16)  scale=2^-15  rndmethod=Unbiased  factor=1  satmethod=Symmetric  shift_vec=[0 1 2 -1]  value=2  inPortNames=['s '; 'd0'; 'd1'; 'd2'; 'd3'; 'd4'; 'd5'; 'd6'; 'd7'; 'd8'; 'd9';]  outPortNames=[' ']  dspbaimage=dspba_prim_tall.svg  text=fprintf('%s', primtype);  style=Optimised  visibilities=1032  version=20211007
  Mux3 : Mux  Inputs=8
  Real-Imag to Complex{,1..3} (4 alike) : RealImagToComplex
  RegField : DSPBAModelBus/RegField  reg_name=DUC_LINEUP_param.HB_Bypass  reg_rwmode=Read/Write  reg_msb=15  reg_lsb=0  reg_mode=Specify via dialog  reg_type=ufix(16)  reg_scale=2^-0  reg_init=0  reg_desc=Description of what is stored in this field  reg_modal=off  reg_desc0=0  reg_desc1=0  reg_desc2=0  reg_desc3=0  reg_desc4=0  reg_desc5=0  reg_desc6=0  reg_desc7=0  reg_addr=4  SampleTime=-1  version=20090407
  SampleDelay : DSPBAPrim/SampleDelay  primtype=sampdelay  nInputs=1  nOutputs=1  omode=Inherit via internal rule  otype=sfix(16)  scale=2^-15  rndmethod=Unbiased  factor=1  satmethod=Symmetric  shift_vec=[0 1 2 -1]  floatPrecision=float32_m23  value=1  inPortNames=[' '; ' ';]  outPortNames=[' ']  dspbaimage=dspba_prim.svg  text=dpoly(1, eye(1,value+1), 'z')  style=Optimised  visibilities=8 + 1024 + 2^17 + 2^18  flexible=off  slackgroup=0  augmented=0  version=20211007  advOptions=[]
  SynInfo : DSPBAPrim/SynthesisInfo  primtype=synthinfo  nInputs=0  nOutputs=0  omode=Inherit via internal rule  otype=sfix(16)  scale=2^-15  rndmethod=Truncate  factor=1  satmethod=Symmetric  shift_vec=[0 1 2 -1]  value=99  inPortNames=[' '; ' ';]  outPortNames=[' ']  dspbaimage=dspba_prim_ctrl.jpg  text=fprintf('Style=%s', style);  style=Scheduled  visibilities=2^17+2^18+2^19+2^20+2^21+2^22+2^23+2^24  constraintPair=None  constraintRelation=>  constraintLimit=4  modelRefSign=+  modelRef=''  showSchedule=off  simulationMode=Use Global Value  resetMinimization=Off  version=20220106
  dout : Outport
  vout : Outport  Port=2
  cout : Outport  Port=3
  wires:
  Channel_out_HC_Bypass/2 -> cout/1
  Channel_out_HC_Bypass/1 -> vout/1
  Channel_out_HC_Bypass/3 -> dout/1
  Channel_In1_HB_Bypass/2 -> Mux2/3
  Channel_In_HB_Bypass/3 -> Mux/2
  Channel_In_HB_Bypass/1 -> Mux1/2
  Channel_In_HB_Bypass/2 -> Mux2/2
  Channel_In1_HB_Bypass/1 -> Mux1/3
  SampleDelay/1 -> BitExtract1/1
  din_intp_out/1 -> Channel_In_HB_Bypass/3
  din_intp_in/1 -> Channel_In1_HB_Bypass/3
  vin_intp_out/1 -> Channel_In_HB_Bypass/1
  cin_intp_in/1 -> Channel_In1_HB_Bypass/2
  cin_intp_out/1 -> Channel_In_HB_Bypass/2
  vin_intp_in/1 -> Channel_In1_HB_Bypass/1
  Mux/1 -> Channel_out_HC_Bypass/3
  Mux1/1 -> Channel_out_HC_Bypass/1
  Mux2/1 -> Channel_out_HC_Bypass/2
  BitExtract1/1 -> Mux2/1, Mux1/1, Mux/1
  RegField/1 -> SampleDelay/1
  Channel_In1_HB_Bypass/3 -> Demux/1
  Demux/1 -> Mux3/1
  Demux/2 -> Mux3/2
  Demux/4 -> Mux3/4
  Demux/3 -> Mux3/3
  Constant2/1 -> Real-Imag to Complex/1
  Real-Imag to Complex/1 -> Mux3/5
  Constant1/1 -> Real-Imag to Complex/2
  Real-Imag to Complex1/1 -> Mux3/6
  Real-Imag to Complex2/1 -> Mux3/7
  Real-Imag to Complex3/1 -> Mux3/8
  Constant3/1 -> Real-Imag to Complex1/1
  Constant4/1 -> Real-Imag to Complex1/2
  Constant5/1 -> Real-Imag to Complex2/1
  Constant6/1 -> Real-Imag to Complex2/2
  Constant7/1 -> Real-Imag to Complex3/1
  Constant8/1 -> Real-Imag to Complex3/2
  Mux3/1 -> Mux/3

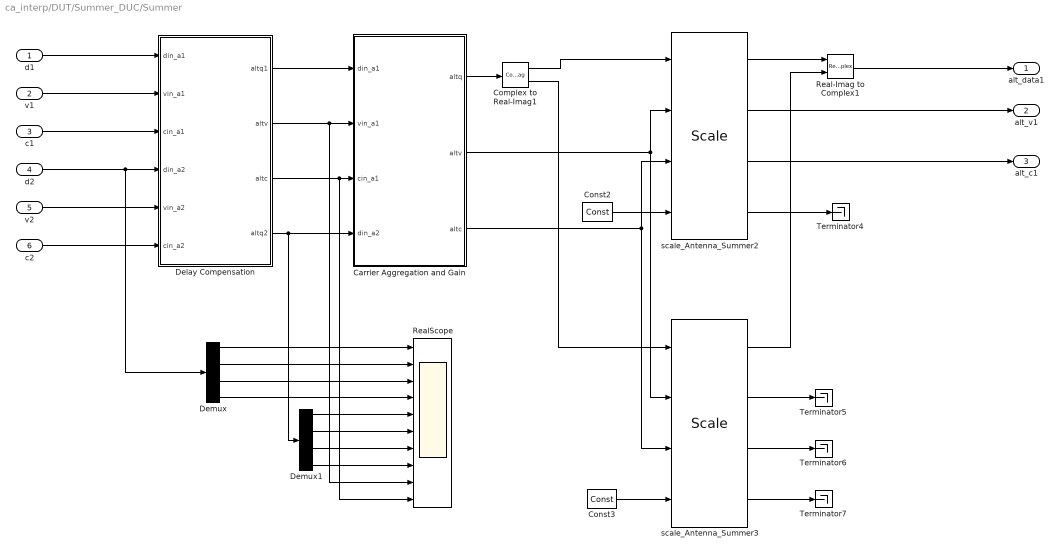
== system ca_interp/DUT/Summer_DUC/Summer ==
  d1 : Inport
  v1 : Inport  Port=2
  c1 : Inport  Port=3
  d2 : Inport  Port=4
  v2 : Inport  Port=5
  c2 : Inport  Port=6
  Carrier Aggregation and Gain : Subsystem
  Complex to Real-Imag1 : ComplexToRealImag
  Const2 : DSPBAPrim/Const  primtype=const  nInputs=0  nOutputs=1  omode=Inherit via internal rule  otype=sfix(16)  scale=2^-15  rndmethod=Unbiased  factor=1  satmethod=Symmetric  shift_vec=[0 1 2 -1]  value=0  inPortNames=['+'; '+';]  outPortNames=[' ']  dspbaimage=dspba_prim.svg  text=fprintf('%s', num2str(value));  style=Optimised  visibilities=8 + 1024  floatPrecision=float32_m23  warnSaturation=on  version=20211007  SampleTime=inf
  Const3 : DSPBAPrim/Const  primtype=const  nInputs=0  nOutputs=1  omode=Inherit via internal rule  otype=sfix(16)  scale=2^-15  rndmethod=Unbiased  factor=1  satmethod=Symmetric  shift_vec=[0 1 2 -1]  value=0  inPortNames=['+'; '+';]  outPortNames=[' ']  dspbaimage=dspba_prim.svg  text=fprintf('%s', num2str(value));  style=Optimised  visibilities=8 + 1024  floatPrecision=float32_m23  warnSaturation=on  version=20211007  SampleTime=inf
  Delay Compensation : Subsystem
  Demux : Demux
  Demux1 : Demux
  Real-Imag to Complex1 : RealImagToComplex
  RealScope : Scope  NumInputPorts=10
  Terminator{4..7} (4 alike) : Terminator
  scale_Antenna_Summer2 : DSPBABase/Scale  otype=sfix(output_word_length)  scale=2^-output_fraction_length  rndmethod=Biased  factor=Summer_Multiplication_fact  satmethod=None  shift_vec=Summer_left_shift_fact  latency=2  simulationMode=Use Global Value  version=20090407
      settings: AttributesFormatString=%<latency>
  scale_Antenna_Summer3 : DSPBABase/Scale  otype=sfix(output_word_length)  scale=2^-output_fraction_length  rndmethod=Biased  factor=Summer_Multiplication_fact  satmethod=None  shift_vec=Summer_left_shift_fact  latency=2  simulationMode=Use Global Value  version=20090407
  alt_data1 : Outport
  alt_v1 : Outport  Port=2
  alt_c1 : Outport  Port=3
  wires:
  Carrier Aggregation and Gain/1(altq) -> Complex to Real-Imag1/1
  Complex to Real-Imag1/1 -> scale_Antenna_Summer2/1
  Const3/1 -> scale_Antenna_Summer3/4
  scale_Antenna_Summer3/4 -> Terminator7/1
  scale_Antenna_Summer2/1 -> Real-Imag to Complex1/1
  scale_Antenna_Summer3/2 -> Terminator5/1
  scale_Antenna_Summer2/4 -> Terminator4/1
  scale_Antenna_Summer3/1 -> Real-Imag to Complex1/2
  Carrier Aggregation and Gain/3(altc) -> scale_Antenna_Summer2/3, scale_Antenna_Summer3/3
  Const2/1 -> scale_Antenna_Summer2/4
  Carrier Aggregation and Gain/2(altv) -> scale_Antenna_Summer2/2, scale_Antenna_Summer3/2
  scale_Antenna_Summer3/3 -> Terminator6/1
  Complex to Real-Imag1/2 -> scale_Antenna_Summer3/1
  scale_Antenna_Summer2/3 -> alt_c1/1
  scale_Antenna_Summer2/2 -> alt_v1/1
  Real-Imag to Complex1/1 -> alt_data1/1
  Delay Compensation/1(altq1) -> Carrier Aggregation and Gain/1(din_a1)
  Delay Compensation/2(altv) -> RealScope/9, Carrier Aggregation and Gain/2(vin_a1)
  Delay Compensation/3(altc) -> RealScope/10, Carrier Aggregation and Gain/3(cin_a1)
  Delay Compensation/4(altq2) -> Demux1/1, Carrier Aggregation and Gain/4(din_a2)
  d1/1 -> Delay Compensation/1(din_a1)
  v1/1 -> Delay Compensation/2(vin_a1)
  c1/1 -> Delay Compensation/3(cin_a1)
  d2/1 -> Demux/1, Delay Compensation/4(din_a2)
  v2/1 -> Delay Compensation/5(vin_a2)
  c2/1 -> Delay Compensation/6(cin_a2)
  Demux/4 -> RealScope/4
  Demux/3 -> RealScope/3
  Demux/2 -> RealScope/2
  Demux/1 -> RealScope/1
  Demux1/1 -> RealScope/5
  Demux1/2 -> RealScope/6
  Demux1/3 -> RealScope/7
  Demux1/4 -> RealScope/8

== system ca_interp/DUT/Summer_DUC/TraceAntennaData ==
  DataIn : Inport
  ChIn : Inport  Port=2
  Enable : EnablePort
  DucAntDataOut : ToWorkspace  VariableName=PolyPhase0_dOut  SampleTime=-1
  DucAntDataOut1 : ToWorkspace  VariableName=PolyPhase0_cOut  SampleTime=-1
  wires:
  DataIn/1 -> DucAntDataOut/1
  ChIn/1 -> DucAntDataOut1/1

== system ca_interp/DUT/Summer_DUC/TraceAntennaData1 ==
  DataIn : Inport
  ChIn : Inport  Port=2
  Enable : EnablePort
  DucAntDataOut : ToWorkspace  VariableName=PolyPhase0_dIn  SampleTime=-1
  DucAntDataOut1 : ToWorkspace  VariableName=PolyPhase0_cIn  SampleTime=-1
  wires:
  ChIn/1 -> DucAntDataOut1/1
  DataIn/1 -> DucAntDataOut/1

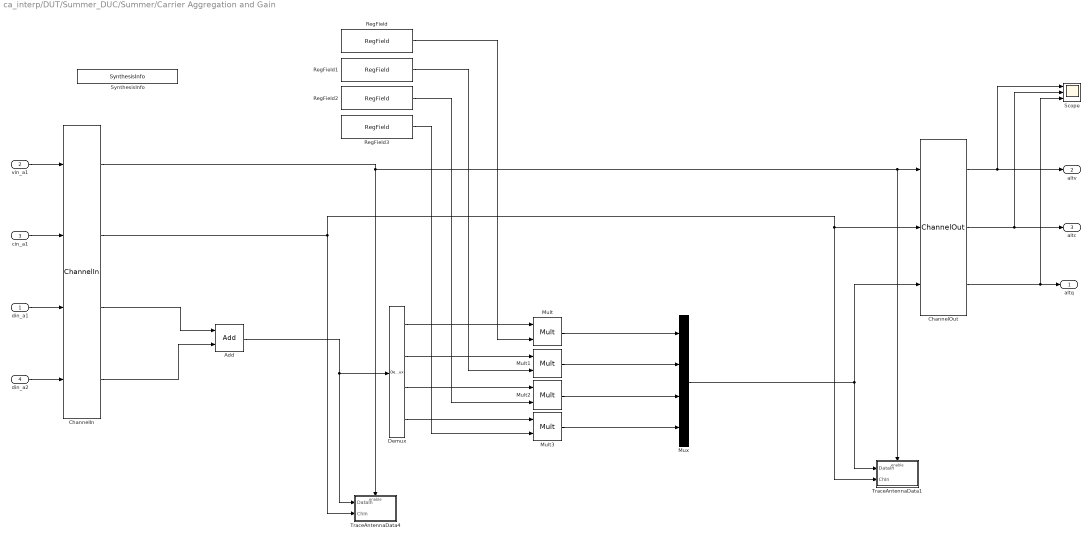
== system ca_interp/DUT/Summer_DUC/Summer/Carrier Aggregation and Gain ==
  din_a1 : Inport
  vin_a1 : Inport  Port=2
  cin_a1 : Inport  Port=3
  din_a2 : Inport  Port=4
  Add : DSPBAPrim/Add  primtype=add  nInputs=evalAionMaskParam(gcb,'value',1)  nOutputs=1  omode=Inherit via internal rule with word growth  otype=sfix(16)  scale=2^-15  rndmethod=Unbiased  factor=1  satmethod=Symmetric  shift_vec=[0 1 2 -1]  value=2  inPortNames=[' '; ' ';]  outPortNames=[' ']  dspbaimage=dspba_prim.svg  text=fprintf('+');  style=Optimised  visibilities=1032+2^17+2^18+2^19  genFPC=off  floatRounding=faithful  advOptions=[]  version=20211007
  ChannelIn : DSPBAPrim/ChannelIn  primtype=channelin  nInputs=dspba_internal_get_channel_ports(gcb)  nOutputs=dspba_internal_get_channel_ports(gcb)  omode=Inherit via internal rule  otype=sfix(16)  scale=2^-15  rndmethod=Unbiased  factor=1  satmethod=Symmetric  shift_vec=[0 1 2 -1]  value=2  inPortNames=['v'; 'c'; '0'; '1'; '2'; '3'; '4'; '5'; '6'; '7'; '8'; '9'; 'A'; 'B'; 'D'; 'E'; 'F'; 'G'; 'H'; 'I'; 'J'; 'K'; 'L'; 'M'; 'N'; 'O'; 'P'; 'Q'; 'R'; 'S'; 'T'; 'U'; 'W'; 'X'; 'Y'; 'Z']  outPortNames=['v'; 'c'; '0'; '1'; '2'; '3'; '4'; '5'; '6'; '7'; '8'; '9'; 'A'; 'B'; 'D'; 'E'; 'F'; 'G'; 'H'; 'I'; 'J'; 'K'; 'L'; 'M'; 'N'; 'O'; 'P'; 'Q'; 'R'; 'S'; 'T'; 'U'; 'W'; 'X'; 'Y'; 'Z']  dspbaimage=dspba_prim_channel_tall.svg  text=fprintf('In');  style=Optimised  dataSignals=2  foldingEnabled=off  channels=1  sampleRate=200  packetBeginPresent=off  packetBeginEnabled=off  visibilities=dspba_ChannelInVis(gcb)  scheduleOrigin=on  version=20211214
  ChannelOut : DSPBAPrim/ChannelOut  primtype=channelout  nInputs=dspba_internal_get_channel_ports(gcb)  nOutputs=dspba_internal_get_channel_ports(gcb)  omode=Inherit via internal rule  otype=sfix(16)  scale=2^-15  rndmethod=Unbiased  factor=1  satmethod=Symmetric  shift_vec=[0 1 2 -1]  value=1  inPortNames=['v'; 'c'; '0'; '1'; '2'; '3'; '4'; '5'; '6'; '7'; '8'; '9'; 'A'; 'B'; 'D'; 'E'; 'F'; 'G'; 'H'; 'I'; 'J'; 'K'; 'L'; 'M'; 'N'; 'O'; 'P'; 'Q'; 'R'; 'S'; 'T'; 'U'; 'W'; 'X'; 'Y'; 'Z']  outPortNames=['v'; 'c'; '0'; '1'; '2'; '3'; '4'; '5'; '6'; '7'; '8'; '9'; 'A'; 'B'; 'D'; 'E'; 'F'; 'G'; 'H'; 'I'; 'J'; 'K'; 'L'; 'M'; 'N'; 'O'; 'P'; 'Q'; 'R'; 'S'; 'T'; 'U'; 'W'; 'X'; 'Y'; 'Z']  dspbaimage=dspba_prim_channel_tall.svg  text=fprintf('Out%s', AdvDSPBChannelOutDisplay(latency));  style=Optimised  dataSignals=1  foldingEnabled=off  channels=1  sampleRate=200  packetBeginPresent=off  packetBeginEnabled=off  visibilities=dspba_ChannelOutVis(gcb)  latency=6  version=20211214
  Demux : Demux
  Mult{,1..3} (4 alike) : DSPBAPrim/Mult  primtype=mult  nInputs=2  nOutputs=1  omode=Inherit via internal rule  otype=sfix(16)  scale=2^-15  rndmethod=Unbiased  factor=1  satmethod=Symmetric  shift_vec=[0 1 2 -1]  value=0  inPortNames=[' '; ' ';]  outPortNames=[' ']  dspbaimage=dspba_prim.svg  text=fprintf('X');  style=Optimised  visibilities=8+2^18+2^19  floatPrecision=float32_m23  floatRounding=correct  advOptions=[]  version=20211007
  Mux : Mux
  RegField : DSPBAModelBus/RegField  reg_name=DUC_Gain_Ant1_offset  reg_rwmode=Read/Write  reg_msb=15  reg_lsb=0  reg_mode=Specify via dialog  reg_type=ufix(16)  reg_scale=2^-13  reg_init=DUC_Gain_Ant1  reg_desc=Digital Gain per Antenna  reg_modal=off  reg_desc0=0  reg_desc1=0  reg_desc2=0  reg_desc3=0  reg_desc4=0  reg_desc5=0  reg_desc6=0  reg_desc7=0  reg_addr=0  SampleTime=-1  version=20090407
  RegField1 : DSPBAModelBus/RegField  reg_name=DUC_Gain_Ant2_offset  reg_rwmode=Read/Write  reg_msb=15  reg_lsb=0  reg_mode=Specify via dialog  reg_type=ufix(16)  reg_scale=2^-13  reg_init=DUC_Gain_Ant2  reg_desc=Digital Gain per Antenna  reg_modal=off  reg_desc0=0  reg_desc1=0  reg_desc2=0  reg_desc3=0  reg_desc4=0  reg_desc5=0  reg_desc6=0  reg_desc7=0  reg_addr=1  SampleTime=-1  version=20090407
  RegField2 : DSPBAModelBus/RegField  reg_name=DUC_Gain_Ant3_offset  reg_rwmode=Read/Write  reg_msb=15  reg_lsb=0  reg_mode=Specify via dialog  reg_type=ufix(16)  reg_scale=2^-13  reg_init=DUC_Gain_Ant3  reg_desc=Digital Gain per Antenna  reg_modal=off  reg_desc0=0  reg_desc1=0  reg_desc2=0  reg_desc3=0  reg_desc4=0  reg_desc5=0  reg_desc6=0  reg_desc7=0  reg_addr=2  SampleTime=-1  version=20090407
  RegField3 : DSPBAModelBus/RegField  reg_name=DUC_Gain_Ant4_offset  reg_rwmode=Read/Write  reg_msb=15  reg_lsb=0  reg_mode=Specify via dialog  reg_type=ufix(16)  reg_scale=2^-13  reg_init=DUC_Gain_Ant4  reg_desc=Digital Gain per Antenna  reg_modal=off  reg_desc0=0  reg_desc1=0  reg_desc2=0  reg_desc3=0  reg_desc4=0  reg_desc5=0  reg_desc6=0  reg_desc7=0  reg_addr=3  SampleTime=-1  version=20090407
  Scope : Scope  NumInputPorts=3
  SynthesisInfo : DSPBAPrim/SynthesisInfo  primtype=synthinfo  nInputs=0  nOutputs=0  omode=Inherit via internal rule  otype=sfix(16)  scale=2^-15  rndmethod=Truncate  factor=1  satmethod=Symmetric  shift_vec=[0 1 2 -1]  value=99  inPortNames=[' '; ' ';]  outPortNames=[' ']  dspbaimage=dspba_prim_ctrl.jpg  text=fprintf('Style=%s', style);  style=Scheduled  visibilities=2^17+2^18+2^19+2^20+2^21+2^22+2^23+2^24  constraintPair=None  constraintRelation=>  constraintLimit=Latency  modelRefSign=+  modelRef=''  showSchedule=off  simulationMode=Use Global Value  resetMinimization=Conditional - On for ChannelIn/Out only  version=20220106
  TraceAntennaData1 : Subsystem  TreatAsAtomicUnit=on
  TraceAntennaData4 : Subsystem  TreatAsAtomicUnit=on
  altq : Outport
  altv : Outport  Port=2
  altc : Outport  Port=3
  wires:
  cin_a1/1 -> ChannelIn/2
  vin_a1/1 -> ChannelIn/1
  din_a1/1 -> ChannelIn/3
  ChannelOut/1 -> Scope/1, altv/1
  ChannelOut/2 -> Scope/2, altc/1
  ChannelOut/3 -> Scope/3, altq/1
  ChannelIn/3 -> Add/1
  ChannelIn/4 -> Add/2
  ChannelIn/1 -> TraceAntennaData4/Enable, TraceAntennaData1/Enable, ChannelOut/1
  Add/1 -> TraceAntennaData4/1(DataIn), Demux/1
  Demux/1 -> Mult/1
  Demux/2 -> Mult1/1
  Demux/3 -> Mult2/1
  Demux/4 -> Mult3/1
  RegField/1 -> Mult/2
  RegField1/1 -> Mult1/2
  RegField2/1 -> Mult2/2
  RegField3/1 -> Mult3/2
  ChannelIn/2 -> TraceAntennaData4/2(ChIn), TraceAntennaData1/2(ChIn), ChannelOut/2
  Mux/1 -> TraceAntennaData1/1(DataIn), ChannelOut/3
  Mult/1 -> Mux/1
  Mult1/1 -> Mux/2
  Mult2/1 -> Mux/3
  Mult3/1 -> Mux/4
  din_a2/1 -> ChannelIn/4
